simulink library "Course_Holes_Lib"  (R2025b)
settings: Solver=ode45  StartTime=0.0  StopTime=10.0  RelTol=1e-3  EnableMultiTasking=on
undefined symbols (not defined in the file): Mini_Golf_Param, X, Y, Z
libraries: Golf_Components_Lib x67, Contact_Forces_Lib x18, sm_lib x12
(part 1 of 2)
Description:
  | Copyright 2015-2025 The MathWorks, Inc.
settings Model: Creator=smiller  LastModifiedBy=smiller
settings SolverCC: AlgebraicLoopSolver=TrustRegion
settings DataIOCC: LimitDataPoints=on  SaveFormat=Array  SignalLoggingSaveFormat=ModelDataLogs  ReturnWorkspaceOutputs=off
settings OptimizationCC: ReuseModelBlockBuffer=off  ExpressionDepthLimit=2147483647.0  LifeSpan=inf
settings DebuggingCC: UnderspecifiedInitializationDetection=Classic  MergeDetectMultiDrivingBlocksExec=none  SolverPrmCheckMsg=warning  FcnCallInpInsideContextMsg=warning  UnconnectedInputMsg=warning  UnconnectedOutputMsg=warning  UnconnectedLineMsg=warning  AllowSymbolicDim=off  StateNameClashWarn=warning  PregeneratedLibrarySubsystemCodeDiagnostic=none  SFUnexpectedBacktrackingDiag=warning  SFNoUnconditionalDefaultTransitionDiag=warning  SFExecutionAtInitializationDiag=none  ArithmeticOperatorsInVariantConditions=warning
settings HardwareCC: ProdBitPerPointer=32.0  ProdBitPerSizeT=32.0  ProdBitPerPtrDiffT=32.0  ProdLargestAtomicFloat=None  ProdIntDivRoundTo=Undefined  ProdEndianess=Unspecified  ProdWordSize=32.0  ProdHWDeviceType=32-bit Generic
settings ModelReferenceCC: EnableRefExpFcnMdlSchedulingChecks=on  PropagateSignalLabelsOutOfModel=off
settings SFSimCC: SimUseLocalCustomCode=off  CustomCodeUndefinedFunction=UseInterfaceOnly
settings RTWCC: RTWUseLocalCustomCode=off  GPUComputeCapability=3.5  DLArmComputeVersion=19.05
settings CodeAppCC: StateflowObjectComments=on
settings GRTTargetCC: TargetLangStandard=C89/C90 (ANSI)
settings ConfigComp: CovMetricSettings=dw  CovSaveCumulativeToWorkspaceVar=on  CovSaveSingleToWorkspaceVar=on  CovExternalEMLEnable=off  CovSFcnEnable=off

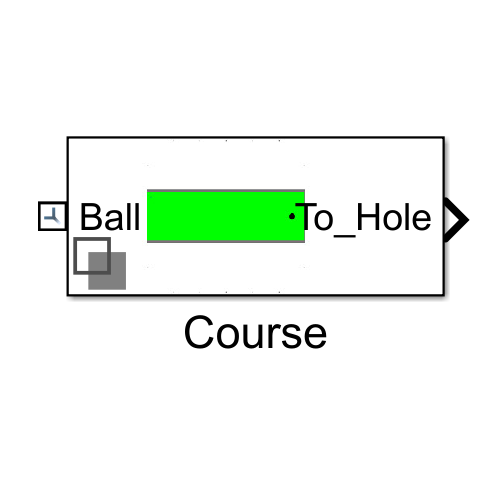
[thumbnail: Simulink's stored preview of the top-level diagram]
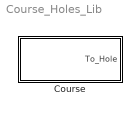
== system Course_Holes_Lib ==
  Course : Subsystem  Variant=on  VariantControlMode=label  LabelModeActiveChoice=Hole_1
      mask Display:
      | blk = CFL_activeVariantBlock(gcb);
      | eval(get_param(blk, 'MaskDisplay'));

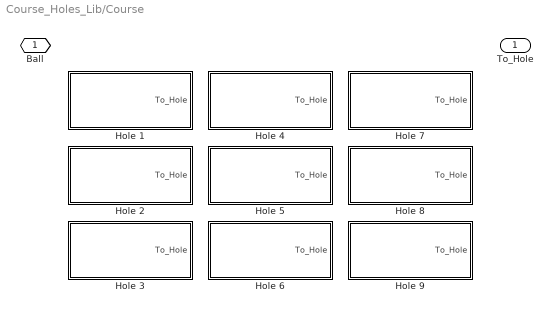
== system Course_Holes_Lib/Course ==
  Hole 1 : Subsystem  VariantControl=Hole_1
      mask Display: image(imread('Hole_1_IMAGE.jpg'));
  Hole 2 : Subsystem  VariantControl=Hole_2
      mask Display: image(imread('Hole_2_IMAGE.jpg'));
  Hole 3 : Subsystem  VariantControl=Hole_3
      mask Display: image(imread('Hole_3_IMAGE.jpg'));
  Hole 4 : Subsystem  VariantControl=Hole_4
      mask Display: image(imread('Hole_4_IMAGE.jpg'));
  Hole 5 : Subsystem  VariantControl=Hole_5
      mask Display: image(imread('Hole_5_IMAGE.jpg'));
  Hole 6 : Subsystem  VariantControl=Hole_6
      mask Display: image(imread('Hole_6_IMAGE.jpg'));
  Hole 7 : Subsystem  VariantControl=Hole_7
      mask Display: image(imread('Hole_7_IMAGE.jpg'));
  Hole 8 : Subsystem  VariantControl=Hole_8
      mask Display: image(imread('Hole_8_IMAGE.jpg'));
  Hole 9 : Subsystem  VariantControl=Hole_9
      mask Display: image(imread('Hole_9_IMAGE.jpg'));
  Ball : PMIOPort  Side=Left
  To_Hole : Outport  VectorParamsAs1DForOutWhenUnconnected=off

== system Course_Holes_Lib/Course/Hole 1 ==
  Back Wall : Golf_Components_Lib/Wall  length=Mini_Golf_Param.Hole_1.Wall_Back.Length  angle=Mini_Golf_Param.Hole_1.Wall_Back.Angle  offset=Mini_Golf_Param.Hole_1.Wall_Back.Offset  height=Mini_Golf_Param.Ball.Radius*2  width=Mini_Golf_Param.Wall.Width  wall_density=Mini_Golf_Param.Wall.Density  ball_radius=Mini_Golf_Param.Ball.Radius  contact_k=Mini_Golf_Param.Wall.Stiffness  contact_b=Mini_Golf_Param.Wall.Damping  low_pass_filt_const=Mini_Golf_Param.Wall.Low_Pass_Filt_Const
  Hole : Golf_Components_Lib/Hole  hole_offset=Mini_Golf_Param.Hole_1.Location  hole_radius=Mini_Golf_Param.Hole.Radius  hole_height=Mini_Golf_Param.Hole.Height  hole_stiffness=Mini_Golf_Param.Hole.Stiffness  hole_damping=Mini_Golf_Param.Hole.Damping  hole_deadzone=Mini_Golf_Param.Hole.Deadzone
  Left Wall : Golf_Components_Lib/Wall  length=Mini_Golf_Param.Hole_1.Wall_Left.Length  angle=Mini_Golf_Param.Hole_1.Wall_Left.Angle  offset=Mini_Golf_Param.Hole_1.Wall_Left.Offset  height=Mini_Golf_Param.Ball.Radius*2  width=Mini_Golf_Param.Wall.Width  wall_density=Mini_Golf_Param.Wall.Density  ball_radius=Mini_Golf_Param.Ball.Radius  contact_k=Mini_Golf_Param.Wall.Stiffness  contact_b=Mini_Golf_Param.Wall.Damping  low_pass_filt_const=Mini_Golf_Param.Wall.Low_Pass_Filt_Const
  Right Wall : Golf_Components_Lib/Wall  length=Mini_Golf_Param.Hole_1.Wall_Right.Length  angle=Mini_Golf_Param.Hole_1.Wall_Right.Angle  offset=Mini_Golf_Param.Hole_1.Wall_Right.Offset  height=Mini_Golf_Param.Ball.Radius*2  width=Mini_Golf_Param.Wall.Width  wall_density=Mini_Golf_Param.Wall.Density  ball_radius=Mini_Golf_Param.Ball.Radius  contact_k=Mini_Golf_Param.Wall.Stiffness  contact_b=Mini_Golf_Param.Wall.Damping  low_pass_filt_const=Mini_Golf_Param.Wall.Low_Pass_Filt_Const
  Surface : Golf_Components_Lib/Surface  width=Mini_Golf_Param.Hole_1.Surface_1.Width  length=Mini_Golf_Param.Hole_1.Surface_1.Length  offset=Mini_Golf_Param.Hole_1.Surface_1.Offset  height=Mini_Golf_Param.Surface_Height
  World Frame : sm_lib/Frames and Transforms/World Frame
  Ball : PMIOPort  Side=Left
  To_Hole : Outport  VectorParamsAs1DForOutWhenUnconnected=off
  wires:
  Hole/1 -> To_Hole/1
  connections:
  Surface/RConn1 -- World Frame/RConn1 -- Hole/RConn1 -- Left Wall/LConn1 -- Back Wall/LConn1 -- Right Wall/LConn1
  Hole/LConn1 -- Right Wall/RConn1 -- Back Wall/RConn1 -- Ball/RConn1 -- Left Wall/RConn1

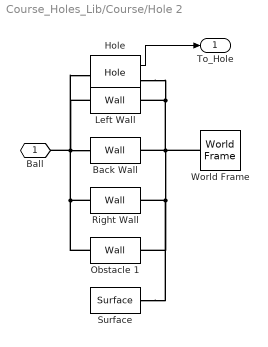
== system Course_Holes_Lib/Course/Hole 2 ==
  Back Wall : Golf_Components_Lib/Wall  length=Mini_Golf_Param.Hole_2.Wall_Back.Length  angle=Mini_Golf_Param.Hole_2.Wall_Back.Angle  offset=Mini_Golf_Param.Hole_2.Wall_Back.Offset  height=Mini_Golf_Param.Ball.Radius*2  width=Mini_Golf_Param.Wall.Width  wall_density=Mini_Golf_Param.Wall.Density  ball_radius=Mini_Golf_Param.Ball.Radius  contact_k=Mini_Golf_Param.Wall.Stiffness  contact_b=Mini_Golf_Param.Wall.Damping  low_pass_filt_const=Mini_Golf_Param.Wall.Low_Pass_Filt_Const
  Hole : Golf_Components_Lib/Hole  hole_offset=Mini_Golf_Param.Hole_2.Location  hole_radius=Mini_Golf_Param.Hole.Radius  hole_height=Mini_Golf_Param.Hole.Height  hole_stiffness=Mini_Golf_Param.Hole.Stiffness  hole_damping=Mini_Golf_Param.Hole.Damping  hole_deadzone=Mini_Golf_Param.Hole.Deadzone
  Left Wall : Golf_Components_Lib/Wall  length=Mini_Golf_Param.Hole_2.Wall_Left.Length  angle=Mini_Golf_Param.Hole_2.Wall_Left.Angle  offset=Mini_Golf_Param.Hole_2.Wall_Left.Offset  height=Mini_Golf_Param.Ball.Radius*2  width=Mini_Golf_Param.Wall.Width  wall_density=Mini_Golf_Param.Wall.Density  ball_radius=Mini_Golf_Param.Ball.Radius  contact_k=Mini_Golf_Param.Wall.Stiffness  contact_b=Mini_Golf_Param.Wall.Damping  low_pass_filt_const=Mini_Golf_Param.Wall.Low_Pass_Filt_Const
  Obstacle 1 : Golf_Components_Lib/Wall  length=Mini_Golf_Param.Hole_2.Wall_Obst1.Length  angle=Mini_Golf_Param.Hole_2.Wall_Obst1.Angle  offset=Mini_Golf_Param.Hole_2.Wall_Obst1.Offset  height=Mini_Golf_Param.Ball.Radius*2  width=Mini_Golf_Param.Wall.Width  wall_density=Mini_Golf_Param.Wall.Density  ball_radius=Mini_Golf_Param.Ball.Radius  contact_k=Mini_Golf_Param.Wall.Stiffness  contact_b=Mini_Golf_Param.Wall.Damping  low_pass_filt_const=Mini_Golf_Param.Wall.Low_Pass_Filt_Const
  Right Wall : Golf_Components_Lib/Wall  length=Mini_Golf_Param.Hole_2.Wall_Right.Length  angle=Mini_Golf_Param.Hole_2.Wall_Right.Angle  offset=Mini_Golf_Param.Hole_2.Wall_Right.Offset  height=Mini_Golf_Param.Ball.Radius*2  width=Mini_Golf_Param.Wall.Width  wall_density=Mini_Golf_Param.Wall.Density  ball_radius=Mini_Golf_Param.Ball.Radius  contact_k=Mini_Golf_Param.Wall.Stiffness  contact_b=Mini_Golf_Param.Wall.Damping  low_pass_filt_const=Mini_Golf_Param.Wall.Low_Pass_Filt_Const
  Surface : Golf_Components_Lib/Surface  width=Mini_Golf_Param.Hole_2.Surface_1.Width  length=Mini_Golf_Param.Hole_2.Surface_1.Length  offset=Mini_Golf_Param.Hole_2.Surface_1.Offset  height=Mini_Golf_Param.Surface_Height
  World Frame : sm_lib/Frames and Transforms/World Frame
  Ball : PMIOPort  Side=Left
  To_Hole : Outport  VectorParamsAs1DForOutWhenUnconnected=off
  wires:
  Hole/1 -> To_Hole/1
  connections:
  Right Wall/RConn1 -- Left Wall/RConn1 -- Hole/LConn1 -- Ball/RConn1 -- Back Wall/RConn1 -- Obstacle 1/RConn1
  World Frame/RConn1 -- Surface/RConn1 -- Obstacle 1/LConn1 -- Right Wall/LConn1 -- Back Wall/LConn1 -- Left Wall/LConn1 -- Hole/RConn1

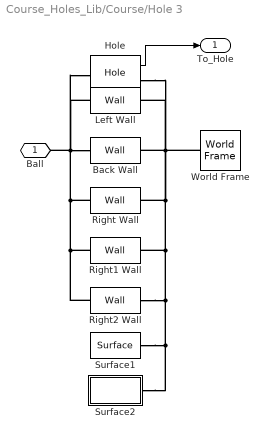
== system Course_Holes_Lib/Course/Hole 3 ==
  Back Wall : Golf_Components_Lib/Wall  length=Mini_Golf_Param.Hole_3.Wall_Back.Length  angle=Mini_Golf_Param.Hole_3.Wall_Back.Angle  offset=Mini_Golf_Param.Hole_3.Wall_Back.Offset  height=Mini_Golf_Param.Ball.Radius*2  width=Mini_Golf_Param.Wall.Width  wall_density=Mini_Golf_Param.Wall.Density  ball_radius=Mini_Golf_Param.Ball.Radius  contact_k=Mini_Golf_Param.Wall.Stiffness  contact_b=Mini_Golf_Param.Wall.Damping  low_pass_filt_const=Mini_Golf_Param.Wall.Low_Pass_Filt_Const
  Hole : Golf_Components_Lib/Hole  hole_offset=Mini_Golf_Param.Hole_3.Location  hole_radius=Mini_Golf_Param.Hole.Radius  hole_height=Mini_Golf_Param.Hole.Height  hole_stiffness=Mini_Golf_Param.Hole.Stiffness  hole_damping=Mini_Golf_Param.Hole.Damping  hole_deadzone=Mini_Golf_Param.Hole.Deadzone
  Left Wall : Golf_Components_Lib/Wall  length=Mini_Golf_Param.Hole_3.Wall_Left.Length  angle=Mini_Golf_Param.Hole_3.Wall_Left.Angle  offset=Mini_Golf_Param.Hole_3.Wall_Left.Offset  height=Mini_Golf_Param.Ball.Radius*2  width=Mini_Golf_Param.Wall.Width  wall_density=Mini_Golf_Param.Wall.Density  ball_radius=Mini_Golf_Param.Ball.Radius  contact_k=Mini_Golf_Param.Wall.Stiffness  contact_b=Mini_Golf_Param.Wall.Damping  low_pass_filt_const=Mini_Golf_Param.Wall.Low_Pass_Filt_Const
  Right Wall : Golf_Components_Lib/Wall  length=Mini_Golf_Param.Hole_3.Wall_Right.Length  angle=Mini_Golf_Param.Hole_3.Wall_Right.Angle  offset=Mini_Golf_Param.Hole_3.Wall_Right.Offset  height=Mini_Golf_Param.Ball.Radius*2  width=Mini_Golf_Param.Wall.Width  wall_density=Mini_Golf_Param.Wall.Density  ball_radius=Mini_Golf_Param.Ball.Radius  contact_k=Mini_Golf_Param.Wall.Stiffness  contact_b=Mini_Golf_Param.Wall.Damping  low_pass_filt_const=Mini_Golf_Param.Wall.Low_Pass_Filt_Const
  Right1 Wall : Golf_Components_Lib/Wall  length=Mini_Golf_Param.Hole_3.Wall_Right1.Length  angle=Mini_Golf_Param.Hole_3.Wall_Right1.Angle  offset=Mini_Golf_Param.Hole_3.Wall_Right1.Offset  height=Mini_Golf_Param.Ball.Radius*2  width=Mini_Golf_Param.Wall.Width  wall_density=Mini_Golf_Param.Wall.Density  ball_radius=Mini_Golf_Param.Ball.Radius  contact_k=Mini_Golf_Param.Wall.Stiffness  contact_b=Mini_Golf_Param.Wall.Damping  low_pass_filt_const=Mini_Golf_Param.Wall.Low_Pass_Filt_Const
  Right2 Wall : Golf_Components_Lib/Wall  length=Mini_Golf_Param.Hole_3.Wall_Right2.Length  angle=Mini_Golf_Param.Hole_3.Wall_Right2.Angle  offset=Mini_Golf_Param.Hole_3.Wall_Right2.Offset  height=Mini_Golf_Param.Ball.Radius*2  width=Mini_Golf_Param.Wall.Width  wall_density=Mini_Golf_Param.Wall.Density  ball_radius=Mini_Golf_Param.Ball.Radius  contact_k=Mini_Golf_Param.Wall.Stiffness  contact_b=Mini_Golf_Param.Wall.Damping  low_pass_filt_const=Mini_Golf_Param.Wall.Low_Pass_Filt_Const
  Surface1 : Golf_Components_Lib/Surface  width=Mini_Golf_Param.Hole_3.Surface_1.Width  length=Mini_Golf_Param.Hole_3.Surface_1.Length  offset=Mini_Golf_Param.Hole_3.Surface_1.Offset  height=Mini_Golf_Param.Surface_Height
  Surface2 : Subsystem  mask(Square Surface Patch for Golf Course){width=Mini_Golf_Param.Hole_3.Surface_2.Width, length=Mini_Golf_Param.Hole_3.Surface_2.Length, offset=Mini_Golf_Param.Hole_3.Surface_2.Offset, height=Mini_Golf_Param.Surface_Height}
      mask prompts: width "Surface Width (m)"; length "Surface Length (m)"; offset "Surface Offset (m)"; height "Surface Thickness(m)"
      mask help: Creates a square surface patch for golf course. All parameters are relative to the frame that is connected to the port.
  World Frame : sm_lib/Frames and Transforms/World Frame
  Ball : PMIOPort  Side=Left
  To_Hole : Outport  VectorParamsAs1DForOutWhenUnconnected=off
  wires:
  Hole/1 -> To_Hole/1
  connections:
  Surface1/RConn1 -- Surface2/RConn1 -- Right2 Wall/LConn1 -- Hole/RConn1 -- Left Wall/LConn1 -- Back Wall/LConn1 -- World Frame/RConn1 -- Right Wall/LConn1 -- Right1 Wall/LConn1
  Right1 Wall/RConn1 -- Right2 Wall/RConn1 -- Back Wall/RConn1 -- Ball/RConn1 -- Hole/LConn1 -- Left Wall/RConn1 -- Right Wall/RConn1

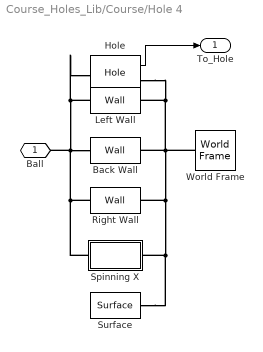
== system Course_Holes_Lib/Course/Hole 4 ==
  Back Wall : Golf_Components_Lib/Wall  length=Mini_Golf_Param.Hole_1.Wall_Back.Length  angle=Mini_Golf_Param.Hole_1.Wall_Back.Angle  offset=Mini_Golf_Param.Hole_1.Wall_Back.Offset  height=Mini_Golf_Param.Ball.Radius*2  width=Mini_Golf_Param.Wall.Width  wall_density=Mini_Golf_Param.Wall.Density  ball_radius=Mini_Golf_Param.Ball.Radius  contact_k=Mini_Golf_Param.Wall.Stiffness  contact_b=Mini_Golf_Param.Wall.Damping  low_pass_filt_const=Mini_Golf_Param.Wall.Low_Pass_Filt_Const
  Hole : Golf_Components_Lib/Hole  hole_offset=Mini_Golf_Param.Hole_1.Location  hole_radius=Mini_Golf_Param.Hole.Radius  hole_height=Mini_Golf_Param.Hole.Height  hole_stiffness=Mini_Golf_Param.Hole.Stiffness  hole_damping=Mini_Golf_Param.Hole.Damping  hole_deadzone=Mini_Golf_Param.Hole.Deadzone
  Left Wall : Golf_Components_Lib/Wall  length=Mini_Golf_Param.Hole_1.Wall_Left.Length  angle=Mini_Golf_Param.Hole_1.Wall_Left.Angle  offset=Mini_Golf_Param.Hole_1.Wall_Left.Offset  height=Mini_Golf_Param.Ball.Radius*2  width=Mini_Golf_Param.Wall.Width  wall_density=Mini_Golf_Param.Wall.Density  ball_radius=Mini_Golf_Param.Ball.Radius  contact_k=Mini_Golf_Param.Wall.Stiffness  contact_b=Mini_Golf_Param.Wall.Damping  low_pass_filt_const=Mini_Golf_Param.Wall.Low_Pass_Filt_Const
  Right Wall : Golf_Components_Lib/Wall  length=Mini_Golf_Param.Hole_1.Wall_Right.Length  angle=Mini_Golf_Param.Hole_1.Wall_Right.Angle  offset=Mini_Golf_Param.Hole_1.Wall_Right.Offset  height=Mini_Golf_Param.Ball.Radius*2  width=Mini_Golf_Param.Wall.Width  wall_density=Mini_Golf_Param.Wall.Density  ball_radius=Mini_Golf_Param.Ball.Radius  contact_k=Mini_Golf_Param.Wall.Stiffness  contact_b=Mini_Golf_Param.Wall.Damping  low_pass_filt_const=Mini_Golf_Param.Wall.Low_Pass_Filt_Const
  Spinning X : Subsystem
  Surface : Golf_Components_Lib/Surface  width=Mini_Golf_Param.Hole_4.Surface_1.Width  length=Mini_Golf_Param.Hole_4.Surface_1.Length  offset=Mini_Golf_Param.Hole_4.Surface_1.Offset  height=Mini_Golf_Param.Surface_Height
  World Frame : sm_lib/Frames and Transforms/World Frame
  Ball : PMIOPort  Side=Left
  To_Hole : Outport  VectorParamsAs1DForOutWhenUnconnected=off
  wires:
  Hole/1 -> To_Hole/1
  connections:
  Spinning X/LConn1 -- Right Wall/RConn1 -- Left Wall/RConn1 -- Hole/LConn1 -- Ball/RConn1 -- Back Wall/RConn1
  Back Wall/LConn1 -- Left Wall/LConn1 -- Hole/RConn1 -- World Frame/RConn1 -- Right Wall/LConn1 -- Spinning X/RConn1 -- Surface/RConn1

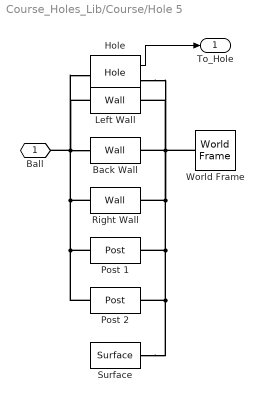
== system Course_Holes_Lib/Course/Hole 5 ==
  Back Wall : Golf_Components_Lib/Wall  length=Mini_Golf_Param.Hole_5.Wall_Back.Length  angle=Mini_Golf_Param.Hole_5.Wall_Back.Angle  offset=Mini_Golf_Param.Hole_5.Wall_Back.Offset  height=Mini_Golf_Param.Ball.Radius*2  width=Mini_Golf_Param.Wall.Width  wall_density=Mini_Golf_Param.Wall.Density  ball_radius=Mini_Golf_Param.Ball.Radius  contact_k=Mini_Golf_Param.Wall.Stiffness  contact_b=Mini_Golf_Param.Wall.Damping  low_pass_filt_const=Mini_Golf_Param.Wall.Low_Pass_Filt_Const
  Hole : Golf_Components_Lib/Hole  hole_offset=Mini_Golf_Param.Hole_5.Location  hole_radius=Mini_Golf_Param.Hole.Radius  hole_height=Mini_Golf_Param.Hole.Height  hole_stiffness=Mini_Golf_Param.Hole.Stiffness  hole_damping=Mini_Golf_Param.Hole.Damping  hole_deadzone=Mini_Golf_Param.Hole.Deadzone
  Left Wall : Golf_Components_Lib/Wall  length=Mini_Golf_Param.Hole_5.Wall_Left.Length  angle=Mini_Golf_Param.Hole_5.Wall_Left.Angle  offset=Mini_Golf_Param.Hole_5.Wall_Left.Offset  height=Mini_Golf_Param.Ball.Radius*2  width=Mini_Golf_Param.Wall.Width  wall_density=Mini_Golf_Param.Wall.Density  ball_radius=Mini_Golf_Param.Ball.Radius  contact_k=Mini_Golf_Param.Wall.Stiffness  contact_b=Mini_Golf_Param.Wall.Damping  low_pass_filt_const=Mini_Golf_Param.Wall.Low_Pass_Filt_Const
  Post 1 : Golf_Components_Lib/Post  width=Mini_Golf_Param.Hole_5.Post_1.Diameter  height=Mini_Golf_Param.Ball.Radius*2  offset=Mini_Golf_Param.Hole_5.Post_1.Offset  ball_radius=Mini_Golf_Param.Ball.Radius  contact_k=Mini_Golf_Param.Wall.Stiffness  contact_b=Mini_Golf_Param.Wall.Damping  low_pass_filt_const=Mini_Golf_Param.Wall.Low_Pass_Filt_Const
  Post 2 : Golf_Components_Lib/Post  width=Mini_Golf_Param.Hole_5.Post_2.Diameter  height=Mini_Golf_Param.Ball.Radius*2  offset=Mini_Golf_Param.Hole_5.Post_2.Offset  ball_radius=Mini_Golf_Param.Ball.Radius  contact_k=Mini_Golf_Param.Wall.Stiffness  contact_b=Mini_Golf_Param.Wall.Damping  low_pass_filt_const=Mini_Golf_Param.Wall.Low_Pass_Filt_Const
  Right Wall : Golf_Components_Lib/Wall  length=Mini_Golf_Param.Hole_5.Wall_Right.Length  angle=Mini_Golf_Param.Hole_5.Wall_Right.Angle  offset=Mini_Golf_Param.Hole_5.Wall_Right.Offset  height=Mini_Golf_Param.Ball.Radius*2  width=Mini_Golf_Param.Wall.Width  wall_density=Mini_Golf_Param.Wall.Density  ball_radius=Mini_Golf_Param.Ball.Radius  contact_k=Mini_Golf_Param.Wall.Stiffness  contact_b=Mini_Golf_Param.Wall.Damping  low_pass_filt_const=Mini_Golf_Param.Wall.Low_Pass_Filt_Const
  Surface : Golf_Components_Lib/Surface  width=Mini_Golf_Param.Hole_5.Surface_1.Width  length=Mini_Golf_Param.Hole_5.Surface_1.Length  offset=Mini_Golf_Param.Hole_5.Surface_1.Offset  height=Mini_Golf_Param.Surface_Height
  World Frame : sm_lib/Frames and Transforms/World Frame
  Ball : PMIOPort  Side=Left
  To_Hole : Outport  VectorParamsAs1DForOutWhenUnconnected=off
  wires:
  Hole/1 -> To_Hole/1
  connections:
  Post 1/RConn1 -- Right Wall/RConn1 -- Left Wall/RConn1 -- Hole/LConn1 -- Ball/RConn1 -- Back Wall/RConn1 -- Post 2/RConn1
  Surface/RConn1 -- Post 1/LConn1 -- Back Wall/LConn1 -- Left Wall/LConn1 -- Hole/RConn1 -- World Frame/RConn1 -- Right Wall/LConn1 -- Post 2/LConn1

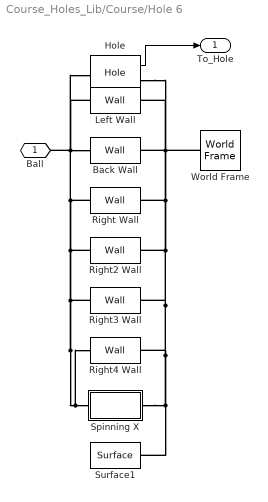
== system Course_Holes_Lib/Course/Hole 6 ==
  Back Wall : Golf_Components_Lib/Wall  length=Mini_Golf_Param.Hole_6.Wall_Back.Length  angle=Mini_Golf_Param.Hole_6.Wall_Back.Angle  offset=Mini_Golf_Param.Hole_6.Wall_Back.Offset  height=Mini_Golf_Param.Ball.Radius*2  width=Mini_Golf_Param.Wall.Width  wall_density=Mini_Golf_Param.Wall.Density  ball_radius=Mini_Golf_Param.Ball.Radius  contact_k=Mini_Golf_Param.Wall.Stiffness  contact_b=Mini_Golf_Param.Wall.Damping  low_pass_filt_const=Mini_Golf_Param.Wall.Low_Pass_Filt_Const
  Hole : Golf_Components_Lib/Hole  hole_offset=Mini_Golf_Param.Hole_6.Location  hole_radius=Mini_Golf_Param.Hole.Radius  hole_height=Mini_Golf_Param.Hole.Height  hole_stiffness=Mini_Golf_Param.Hole.Stiffness  hole_damping=Mini_Golf_Param.Hole.Damping  hole_deadzone=Mini_Golf_Param.Hole.Deadzone
  Left Wall : Golf_Components_Lib/Wall  length=Mini_Golf_Param.Hole_6.Wall_Left.Length  angle=Mini_Golf_Param.Hole_6.Wall_Left.Angle  offset=Mini_Golf_Param.Hole_6.Wall_Left.Offset  height=Mini_Golf_Param.Ball.Radius*2  width=Mini_Golf_Param.Wall.Width  wall_density=Mini_Golf_Param.Wall.Density  ball_radius=Mini_Golf_Param.Ball.Radius  contact_k=Mini_Golf_Param.Wall.Stiffness  contact_b=Mini_Golf_Param.Wall.Damping  low_pass_filt_const=Mini_Golf_Param.Wall.Low_Pass_Filt_Const
  Right Wall : Golf_Components_Lib/Wall  length=Mini_Golf_Param.Hole_6.Wall_Right.Length  angle=Mini_Golf_Param.Hole_6.Wall_Right.Angle  offset=Mini_Golf_Param.Hole_6.Wall_Right.Offset  height=Mini_Golf_Param.Ball.Radius*2  width=Mini_Golf_Param.Wall.Width  wall_density=Mini_Golf_Param.Wall.Density  ball_radius=Mini_Golf_Param.Ball.Radius  contact_k=Mini_Golf_Param.Wall.Stiffness  contact_b=Mini_Golf_Param.Wall.Damping  low_pass_filt_const=Mini_Golf_Param.Wall.Low_Pass_Filt_Const
  Right2 Wall : Golf_Components_Lib/Wall  length=Mini_Golf_Param.Hole_6.Wall_Right2.Length  angle=Mini_Golf_Param.Hole_6.Wall_Right2.Angle  offset=Mini_Golf_Param.Hole_6.Wall_Right2.Offset  height=Mini_Golf_Param.Ball.Radius*2  width=Mini_Golf_Param.Wall.Width  wall_density=Mini_Golf_Param.Wall.Density  ball_radius=Mini_Golf_Param.Ball.Radius  contact_k=Mini_Golf_Param.Wall.Stiffness  contact_b=Mini_Golf_Param.Wall.Damping  low_pass_filt_const=Mini_Golf_Param.Wall.Low_Pass_Filt_Const
  Right3 Wall : Golf_Components_Lib/Wall  length=Mini_Golf_Param.Hole_6.Wall_Right3.Length  angle=Mini_Golf_Param.Hole_6.Wall_Right3.Angle  offset=Mini_Golf_Param.Hole_6.Wall_Right3.Offset  height=Mini_Golf_Param.Ball.Radius*2  width=Mini_Golf_Param.Wall.Width  wall_density=Mini_Golf_Param.Wall.Density  ball_radius=Mini_Golf_Param.Ball.Radius  contact_k=Mini_Golf_Param.Wall.Stiffness  contact_b=Mini_Golf_Param.Wall.Damping  low_pass_filt_const=Mini_Golf_Param.Wall.Low_Pass_Filt_Const
  Right4 Wall : Golf_Components_Lib/Wall  length=Mini_Golf_Param.Hole_6.Wall_Right4.Length  angle=Mini_Golf_Param.Hole_6.Wall_Right4.Angle  offset=Mini_Golf_Param.Hole_6.Wall_Right4.Offset  height=Mini_Golf_Param.Ball.Radius*2  width=Mini_Golf_Param.Wall.Width  wall_density=Mini_Golf_Param.Wall.Density  ball_radius=Mini_Golf_Param.Ball.Radius  contact_k=Mini_Golf_Param.Wall.Stiffness  contact_b=Mini_Golf_Param.Wall.Damping  low_pass_filt_const=Mini_Golf_Param.Wall.Low_Pass_Filt_Const
  Spinning X : Subsystem
  Surface1 : Golf_Components_Lib/Surface  width=Mini_Golf_Param.Hole_6.Surface_1.Width  length=Mini_Golf_Param.Hole_6.Surface_1.Length  offset=Mini_Golf_Param.Hole_6.Surface_1.Offset  height=Mini_Golf_Param.Surface_Height
  World Frame : sm_lib/Frames and Transforms/World Frame
  Ball : PMIOPort  Side=Left
  To_Hole : Outport  VectorParamsAs1DForOutWhenUnconnected=off
  wires:
  Hole/1 -> To_Hole/1
  connections:
  Spinning X/LConn1 -- Right3 Wall/RConn1 -- Right2 Wall/RConn1 -- Right Wall/RConn1 -- Left Wall/RConn1 -- Hole/LConn1 -- Ball/RConn1 -- Back Wall/RConn1 -- Right4 Wall/RConn1
  Spinning X/RConn1 -- Right2 Wall/LConn1 -- Right Wall/LConn1 -- World Frame/RConn1 -- Back Wall/LConn1 -- Left Wall/LConn1 -- Hole/RConn1 -- Right3 Wall/LConn1 -- Right4 Wall/LConn1 -- Surface1/RConn1

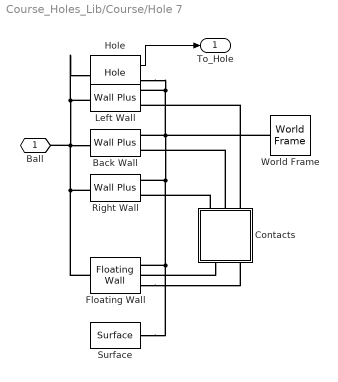
== system Course_Holes_Lib/Course/Hole 7 ==
  Back Wall : Golf_Components_Lib/Wall Plus  length=Mini_Golf_Param.Hole_7.Wall_Back.Length  angle=Mini_Golf_Param.Hole_7.Wall_Back.Angle  offset=Mini_Golf_Param.Hole_7.Wall_Back.Offset  height=Mini_Golf_Param.Ball.Radius*2  width=Mini_Golf_Param.Wall.Width  ball_radius=Mini_Golf_Param.Ball.Radius  contact_k=Mini_Golf_Param.Wall.Stiffness  contact_b=Mini_Golf_Param.Wall.Damping  low_pass_filt_const=Mini_Golf_Param.Wall.Low_Pass_Filt_Const
  Contacts : Subsystem
  Floating Wall : Golf_Components_Lib/Floating Wall  length=Mini_Golf_Param.Hole_7.Wall_Obst1.Length  angle=Mini_Golf_Param.Hole_7.Wall_Obst1.Angle  offset=Mini_Golf_Param.Hole_7.Wall_Obst1.Offset  height=Mini_Golf_Param.Ball.Radius*2  width=Mini_Golf_Param.Wall.Width  wall_friction=Mini_Golf_Param.Hole_7.Wall_Obst1.Friction  wall_rot_friction=Mini_Golf_Param.Hole_7.Wall_Obst1.Rot_Friction  ball_radius=Mini_Golf_Param.Ball.Radius  contact_k=Mini_Golf_Param.Wall.Stiffness  contact_b=Mini_Golf_Param.Wall.Damping  low_pass_filt_const=Mini_Golf_Param.Wall.Low_Pass_Filt_Const
  Hole : Golf_Components_Lib/Hole  hole_offset=Mini_Golf_Param.Hole_7.Location  hole_radius=Mini_Golf_Param.Hole.Radius  hole_height=Mini_Golf_Param.Hole.Height  hole_stiffness=Mini_Golf_Param.Hole.Stiffness  hole_damping=Mini_Golf_Param.Hole.Damping  hole_deadzone=Mini_Golf_Param.Hole.Deadzone
  Left Wall : Golf_Components_Lib/Wall Plus  length=Mini_Golf_Param.Hole_7.Wall_Left.Length  angle=Mini_Golf_Param.Hole_7.Wall_Left.Angle  offset=Mini_Golf_Param.Hole_7.Wall_Left.Offset  height=Mini_Golf_Param.Ball.Radius*2  width=Mini_Golf_Param.Wall.Width  ball_radius=Mini_Golf_Param.Ball.Radius  contact_k=Mini_Golf_Param.Wall.Stiffness  contact_b=Mini_Golf_Param.Wall.Damping  low_pass_filt_const=Mini_Golf_Param.Wall.Low_Pass_Filt_Const
  Right Wall : Golf_Components_Lib/Wall Plus  length=Mini_Golf_Param.Hole_7.Wall_Right.Length  angle=Mini_Golf_Param.Hole_7.Wall_Right.Angle  offset=Mini_Golf_Param.Hole_7.Wall_Right.Offset  height=Mini_Golf_Param.Ball.Radius*2  width=Mini_Golf_Param.Wall.Width  ball_radius=Mini_Golf_Param.Ball.Radius  contact_k=Mini_Golf_Param.Wall.Stiffness  contact_b=Mini_Golf_Param.Wall.Damping  low_pass_filt_const=Mini_Golf_Param.Wall.Low_Pass_Filt_Const
  Surface : Golf_Components_Lib/Surface  width=Mini_Golf_Param.Hole_7.Surface_1.Width  length=Mini_Golf_Param.Hole_7.Surface_1.Length  offset=Mini_Golf_Param.Hole_7.Surface_1.Offset  height=Mini_Golf_Param.Surface_Height
  World Frame : sm_lib/Frames and Transforms/World Frame
  Ball : PMIOPort  Side=Left
  To_Hole : Outport  VectorParamsAs1DForOutWhenUnconnected=off
  wires:
  Hole/1 -> To_Hole/1
  connections:
  Right Wall/LConn1 -- Hole/RConn1 -- Left Wall/LConn1 -- World Frame/RConn1 -- Back Wall/LConn1 -- Surface/RConn1 -- Floating Wall/LConn1
  Ball/RConn1 -- Floating Wall/RConn1 -- Right Wall/RConn1 -- Hole/LConn1 -- Left Wall/RConn1 -- Back Wall/RConn1
  Contacts/LConn1 -- Floating Wall/LConn2
  Floating Wall/LConn3 -- Contacts/LConn2
  Contacts/RConn1 -- Right Wall/LConn2
  Contacts/RConn2 -- Back Wall/LConn2
  Contacts/RConn3 -- Left Wall/LConn2

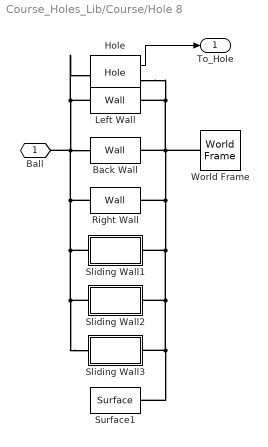
== system Course_Holes_Lib/Course/Hole 8 ==
  Back Wall : Golf_Components_Lib/Wall  length=Mini_Golf_Param.Hole_8.Wall_Back.Length  angle=Mini_Golf_Param.Hole_8.Wall_Back.Angle  offset=Mini_Golf_Param.Hole_8.Wall_Back.Offset  height=Mini_Golf_Param.Ball.Radius*2  width=Mini_Golf_Param.Wall.Width  wall_density=Mini_Golf_Param.Wall.Density  ball_radius=Mini_Golf_Param.Ball.Radius  contact_k=Mini_Golf_Param.Wall.Stiffness  contact_b=Mini_Golf_Param.Wall.Damping  low_pass_filt_const=Mini_Golf_Param.Wall.Low_Pass_Filt_Const
  Hole : Golf_Components_Lib/Hole  hole_offset=Mini_Golf_Param.Hole_8.Location  hole_radius=Mini_Golf_Param.Hole.Radius  hole_height=Mini_Golf_Param.Hole.Height  hole_stiffness=Mini_Golf_Param.Hole.Stiffness  hole_damping=Mini_Golf_Param.Hole.Damping  hole_deadzone=Mini_Golf_Param.Hole.Deadzone
  Left Wall : Golf_Components_Lib/Wall  length=Mini_Golf_Param.Hole_8.Wall_Left.Length  angle=Mini_Golf_Param.Hole_8.Wall_Left.Angle  offset=Mini_Golf_Param.Hole_8.Wall_Left.Offset  height=Mini_Golf_Param.Ball.Radius*2  width=Mini_Golf_Param.Wall.Width  wall_density=Mini_Golf_Param.Wall.Density  ball_radius=Mini_Golf_Param.Ball.Radius  contact_k=Mini_Golf_Param.Wall.Stiffness  contact_b=Mini_Golf_Param.Wall.Damping  low_pass_filt_const=Mini_Golf_Param.Wall.Low_Pass_Filt_Const
  Right Wall : Golf_Components_Lib/Wall  length=Mini_Golf_Param.Hole_8.Wall_Right.Length  angle=Mini_Golf_Param.Hole_8.Wall_Right.Angle  offset=Mini_Golf_Param.Hole_8.Wall_Right.Offset  height=Mini_Golf_Param.Ball.Radius*2  width=Mini_Golf_Param.Wall.Width  wall_density=Mini_Golf_Param.Wall.Density  ball_radius=Mini_Golf_Param.Ball.Radius  contact_k=Mini_Golf_Param.Wall.Stiffness  contact_b=Mini_Golf_Param.Wall.Damping  low_pass_filt_const=Mini_Golf_Param.Wall.Low_Pass_Filt_Const
  Sliding Wall1 : Subsystem
  Sliding Wall2 : Subsystem
  Sliding Wall3 : Subsystem
  Surface1 : Golf_Components_Lib/Surface  width=Mini_Golf_Param.Hole_8.Surface_1.Width  length=Mini_Golf_Param.Hole_8.Surface_1.Length  offset=Mini_Golf_Param.Hole_8.Surface_1.Offset  height=Mini_Golf_Param.Surface_Height
  World Frame : sm_lib/Frames and Transforms/World Frame
  Ball : PMIOPort  Side=Left
  To_Hole : Outport  VectorParamsAs1DForOutWhenUnconnected=off
  wires:
  Hole/1 -> To_Hole/1
  connections:
  Sliding Wall3/LConn1 -- Surface1/RConn1 -- Hole/RConn1 -- Left Wall/LConn1 -- Back Wall/LConn1 -- World Frame/RConn1 -- Right Wall/LConn1 -- Sliding Wall1/LConn1 -- Sliding Wall2/LConn1
  Sliding Wall3/RConn1 -- Back Wall/RConn1 -- Ball/RConn1 -- Hole/LConn1 -- Left Wall/RConn1 -- Right Wall/RConn1 -- Sliding Wall1/RConn1 -- Sliding Wall2/RConn1

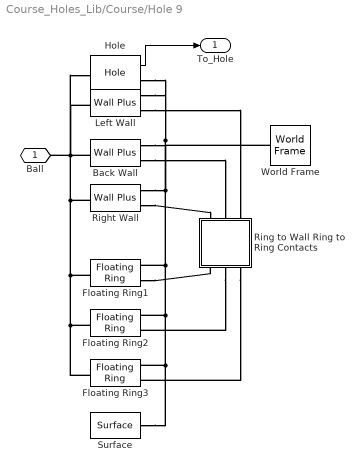
== system Course_Holes_Lib/Course/Hole 9 ==
  Back Wall : Golf_Components_Lib/Wall Plus  length=Mini_Golf_Param.Hole_9.Wall_Back.Length  angle=Mini_Golf_Param.Hole_9.Wall_Back.Angle  offset=Mini_Golf_Param.Hole_9.Wall_Back.Offset  height=Mini_Golf_Param.Ball.Radius*2  width=Mini_Golf_Param.Wall.Width  ball_radius=Mini_Golf_Param.Ball.Radius  contact_k=Mini_Golf_Param.Wall.Stiffness  contact_b=Mini_Golf_Param.Wall.Damping  low_pass_filt_const=Mini_Golf_Param.Wall.Low_Pass_Filt_Const
  Floating Ring1 : Golf_Components_Lib/Floating Ring  extr_xy_data=Mini_Golf_Param.Hole_9.Extr1.Cross_Section_Data  offset=Mini_Golf_Param.Hole_9.Extr1.Offset  height=Mini_Golf_Param.Ball.Radius*2  diameter=Mini_Golf_Param.Hole_9.Extr1.Ring_Outer_Diameter  extr1_friction=Mini_Golf_Param.Hole_9.Extr1.Friction  ball_radius=Mini_Golf_Param.Ball.Radius  contact_k=Mini_Golf_Param.Wall.Stiffness  contact_b=Mini_Golf_Param.Wall.Damping  low_pass_filt_const=Mini_Golf_Param.Wall.Low_Pass_Filt_Const
  Floating Ring2 : Golf_Components_Lib/Floating Ring  extr_xy_data=Mini_Golf_Param.Hole_9.Extr2.Cross_Section_Data  offset=Mini_Golf_Param.Hole_9.Extr2.Offset  height=Mini_Golf_Param.Ball.Radius*2  diameter=Mini_Golf_Param.Hole_9.Extr2.Ring_Outer_Diameter  extr1_friction=Mini_Golf_Param.Hole_9.Extr2.Friction  ball_radius=Mini_Golf_Param.Ball.Radius  contact_k=Mini_Golf_Param.Wall.Stiffness  contact_b=Mini_Golf_Param.Wall.Damping  low_pass_filt_const=Mini_Golf_Param.Wall.Low_Pass_Filt_Const
  Floating Ring3 : Golf_Components_Lib/Floating Ring  extr_xy_data=Mini_Golf_Param.Hole_9.Extr3.Cross_Section_Data  offset=Mini_Golf_Param.Hole_9.Extr3.Offset  height=Mini_Golf_Param.Ball.Radius*2  diameter=Mini_Golf_Param.Hole_9.Extr3.Ring_Outer_Diameter  extr1_friction=Mini_Golf_Param.Hole_9.Extr3.Friction  ball_radius=Mini_Golf_Param.Ball.Radius  contact_k=Mini_Golf_Param.Wall.Stiffness  contact_b=Mini_Golf_Param.Wall.Damping  low_pass_filt_const=Mini_Golf_Param.Wall.Low_Pass_Filt_Const
  Hole : Golf_Components_Lib/Hole  hole_offset=Mini_Golf_Param.Hole_9.Location  hole_radius=Mini_Golf_Param.Hole.Radius  hole_height=Mini_Golf_Param.Hole.Height  hole_stiffness=Mini_Golf_Param.Hole.Stiffness  hole_damping=Mini_Golf_Param.Hole.Damping  hole_deadzone=Mini_Golf_Param.Hole.Deadzone
  Left Wall : Golf_Components_Lib/Wall Plus  length=Mini_Golf_Param.Hole_9.Wall_Left.Length  angle=Mini_Golf_Param.Hole_9.Wall_Left.Angle  offset=Mini_Golf_Param.Hole_9.Wall_Left.Offset  height=Mini_Golf_Param.Ball.Radius*2  width=Mini_Golf_Param.Wall.Width  ball_radius=Mini_Golf_Param.Ball.Radius  contact_k=Mini_Golf_Param.Wall.Stiffness  contact_b=Mini_Golf_Param.Wall.Damping  low_pass_filt_const=Mini_Golf_Param.Wall.Low_Pass_Filt_Const
  Right Wall : Golf_Components_Lib/Wall Plus  length=Mini_Golf_Param.Hole_9.Wall_Right.Length  angle=Mini_Golf_Param.Hole_9.Wall_Right.Angle  offset=Mini_Golf_Param.Hole_9.Wall_Right.Offset  height=Mini_Golf_Param.Ball.Radius*2  width=Mini_Golf_Param.Wall.Width  ball_radius=Mini_Golf_Param.Ball.Radius  contact_k=Mini_Golf_Param.Wall.Stiffness  contact_b=Mini_Golf_Param.Wall.Damping  low_pass_filt_const=Mini_Golf_Param.Wall.Low_Pass_Filt_Const
  Ring to Wall Ring to Ring Contacts : Subsystem
  Surface : Golf_Components_Lib/Surface  width=Mini_Golf_Param.Hole_9.Surface_1.Width  length=Mini_Golf_Param.Hole_9.Surface_1.Length  offset=Mini_Golf_Param.Hole_9.Surface_1.Offset  height=Mini_Golf_Param.Surface_Height
  World Frame : sm_lib/Frames and Transforms/World Frame
  Ball : PMIOPort  Side=Left
  To_Hole : Outport  VectorParamsAs1DForOutWhenUnconnected=off
  wires:
  Hole/1 -> To_Hole/1
  connections:
  Left Wall/LConn2 -- Ring to Wall Ring to Ring Contacts/RConn3
  Back Wall/LConn2 -- Ring to Wall Ring to Ring Contacts/RConn2
  Right Wall/LConn2 -- Ring to Wall Ring to Ring Contacts/RConn1
  Floating Ring1/LConn2 -- Ring to Wall Ring to Ring Contacts/LConn1
  Floating Ring2/RConn1 -- Floating Ring1/RConn1 -- Right Wall/RConn1 -- Back Wall/RConn1 -- Left Wall/RConn1 -- Hole/LConn1 -- Ball/RConn1 -- Floating Ring3/RConn1
  Surface/RConn1 -- Right Wall/LConn1 -- Back Wall/LConn1 -- World Frame/RConn1 -- Left Wall/LConn1 -- Hole/RConn1 -- Floating Ring1/LConn1 -- Floating Ring2/LConn1 -- Floating Ring3/LConn1
  Ring to Wall Ring to Ring Contacts/LConn2 -- Floating Ring2/LConn2
  Ring to Wall Ring to Ring Contacts/LConn3 -- Floating Ring3/LConn2

== system Course_Holes_Lib/Course/Hole 3/Surface2 ==
  Rigid Transform : sm_lib/Frames and Transforms/Rigid Transform  RotationMethod=None  FollAlignAxisA=+X  BaseAlignAxisA=+Y  FollAlignAxisB=+Y  BaseAlignAxisB=+Z  RotationStandardAxis=+Z  RotationAngle=0  RotationAngleUnits=deg  RotationArbitraryAxis=[0 0 1]  RotationSequenceAxes=FollowerAxes  RotationSequence=XYX  RotationSequenceAngles=[0 0 0]  RotationSequenceAnglesUnits=deg  RotationMatrix=[1 0 0; 0 1 0; 0 0 1]  Quaternion=[1 0 0 0]  TranslationMethod=Cartesian  TranslationCartesianOffset=offset  TranslationCartesianOffsetUnits=m  TranslationStandardAxis=+Z  TranslationStandardOffset=0  TranslationStandardOffsetUnits=m  TranslationROffset=0  TranslationROffsetUnits=m  TranslationThetaOffset=0  TranslationThetaOffsetUnits=deg  TranslationZOffset=0  TranslationZOffsetUnits=m
  Surface Patch : sm_lib/Body Elements/Brick Solid  BrickDimensions=[length width height]  BrickDimensionsUnits=m  ExportEntireGeometry=off  InertiaType=CalculateFromGeometry  BasedOnType=Density  Density=1  DensityUnits=kg/(m^3)  Mass=1  MassUnits=kg  CenterOfMass=[0 0 0]  CenterOfMassUnits=m  MomentsOfInertia=[1 1 1]  MomentsOfInertiaUnits=kg*m^2  ProductsOfInertia=[0 0 0]  ProductsOfInertiaUnits=kg*m^2  GraphicType=FromGeometry  MarkerShape=Sphere  MarkerSize=10  GraphicVisPropType=SimpleVisualProperties  GraphicDiffuseColor=[0.0 0.8 0.2]  GraphicOpacity=1.0  GraphicSpecularColor=[0.5 0.5 0.5 1.0]  GraphicAmbientColor=[0.15 0.15 0.15 1.0]  GraphicEmissiveColor=[0.0 0.0 0.0 1.0]  GraphicShininess=75  DoExposeReferenceFrame=on  SerializedFrames=<Frames/>
  Weld Joint : sm_lib/Joints/Weld Joint  JointMode=Normal  CompositeWrenchDir=FollowerOnBase  CompositeWrenchFrame=BaseFrame  SenseConstraintForce=off  SenseConstraintTorque=off  SenseTotalForce=off  SenseTotalTorque=off
  Ref : PMIOPort  Side=Right
  connections:
  Weld Joint/LConn1 -- Ref/RConn1
  Rigid Transform/LConn1 -- Weld Joint/RConn1
  Rigid Transform/RConn1 -- Surface Patch/RConn1

== system Course_Holes_Lib/Course/Hole 4/Spinning X ==
  Spinning Wall : Golf_Components_Lib/Spinning Wall  length=Mini_Golf_Param.Hole_4.Wall_Obst1.Length  angle=Mini_Golf_Param.Hole_4.Wall_Obst1.Angle  offset=Mini_Golf_Param.Hole_4.Wall_Obst1.Offset  ang_spd=Mini_Golf_Param.Hole_4.Obst_Pin.Speed  height=Mini_Golf_Param.Ball.Radius*2  width=Mini_Golf_Param.Wall.Width  wall_density=Mini_Golf_Param.Wall.Density  ball_radius=Mini_Golf_Param.Ball.Radius  contact_k=Mini_Golf_Param.Wall.Stiffness  contact_b=Mini_Golf_Param.Wall.Damping  low_pass_filt_const=Mini_Golf_Param.Wall.Low_Pass_Filt_Const
  Wall : Golf_Components_Lib/Wall  length=Mini_Golf_Param.Hole_4.Wall_Obst2.Length  angle=Mini_Golf_Param.Hole_4.Wall_Obst2.Angle  offset=Mini_Golf_Param.Hole_4.Wall_Obst2.Offset*0  height=Mini_Golf_Param.Ball.Radius*2  width=Mini_Golf_Param.Wall.Width  wall_density=Mini_Golf_Param.Wall.Density  ball_radius=Mini_Golf_Param.Ball.Radius  contact_k=Mini_Golf_Param.Wall.Stiffness  contact_b=Mini_Golf_Param.Wall.Damping  low_pass_filt_const=Mini_Golf_Param.Wall.Low_Pass_Filt_Const
  Ref : PMIOPort  Side=Right
  Ball : PMIOPort  Port=2  Side=Left
  connections:
  Spinning Wall/LConn2 -- Wall/LConn1
  Spinning Wall/RConn1 -- Wall/RConn1 -- Ball/RConn1
  Spinning Wall/LConn1 -- Ref/RConn1

== system Course_Holes_Lib/Course/Hole 6/Spinning X ==
  Spinning Wall : Golf_Components_Lib/Spinning Wall  length=Mini_Golf_Param.Hole_6.Wall_Obst1.Length  angle=Mini_Golf_Param.Hole_6.Wall_Obst1.Angle  offset=Mini_Golf_Param.Hole_6.Wall_Obst1.Offset  ang_spd=Mini_Golf_Param.Hole_6.Obst_Pin.Speed  height=Mini_Golf_Param.Ball.Radius*2  width=Mini_Golf_Param.Wall.Width  wall_density=Mini_Golf_Param.Wall.Density  ball_radius=Mini_Golf_Param.Ball.Radius  contact_k=Mini_Golf_Param.Wall.Stiffness  contact_b=Mini_Golf_Param.Wall.Damping  low_pass_filt_const=Mini_Golf_Param.Wall.Low_Pass_Filt_Const
  Wall : Golf_Components_Lib/Wall  length=Mini_Golf_Param.Hole_6.Wall_Obst2.Length  angle=Mini_Golf_Param.Hole_6.Wall_Obst2.Angle  offset=Mini_Golf_Param.Hole_6.Wall_Obst2.Offset*0  height=Mini_Golf_Param.Ball.Radius*2  width=Mini_Golf_Param.Wall.Width  wall_density=Mini_Golf_Param.Wall.Density  ball_radius=Mini_Golf_Param.Ball.Radius  contact_k=Mini_Golf_Param.Wall.Stiffness  contact_b=Mini_Golf_Param.Wall.Damping  low_pass_filt_const=Mini_Golf_Param.Wall.Low_Pass_Filt_Const
  Ref : PMIOPort  Side=Right
  Ball : PMIOPort  Port=2  Side=Left
  connections:
  Spinning Wall/LConn2 -- Wall/LConn1
  Wall/RConn1 -- Ball/RConn1 -- Spinning Wall/RConn1
  Spinning Wall/LConn1 -- Ref/RConn1

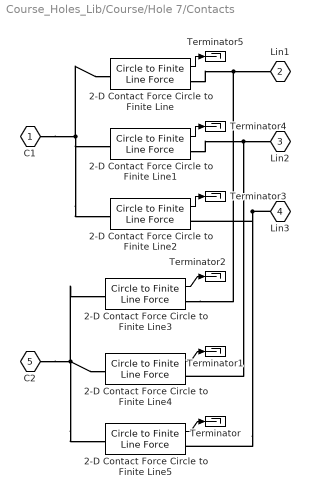
== system Course_Holes_Lib/Course/Hole 7/Contacts ==
  2-D Contact Force Circle to Finite Line : Contact_Forces_Lib/2D/Circle to Finite Line Force  circle_rad=Mini_Golf_Param.Ball.Radius  line_depth=Mini_Golf_Param.Wall.Width/2  line_length=Mini_Golf_Param.Hole_7.Wall_Right.Length  force_law=Linear  k_contact=Mini_Golf_Param.Wall.Stiffness  b_contact=Mini_Golf_Param.Wall.Damping  pen_full_damp_F=1e-4  pen_exponent=1  custom_param_1=1  custom_param_2=1  friction_law=None  mu_kinetic=0.5  mu_static=0.7  v_thr=0.001  vis_on=off  vis_opc_en=0  vis_len_linBz=0.1  vis_len_linBx=0.005  vis_len_cirFz=0.1  vis_len_cirFx=0.005  vis_clr=[0.9 0.2 0.2]  vis_opc=0.7
      settings: SourceProductName=Simscape Multibody Contact Forces Library
  2-D Contact Force Circle to Finite Line1 : Contact_Forces_Lib/2D/Circle to Finite Line Force  circle_rad=Mini_Golf_Param.Ball.Radius  line_depth=Mini_Golf_Param.Wall.Width/2  line_length=Mini_Golf_Param.Hole_7.Wall_Back.Length  force_law=Linear  k_contact=Mini_Golf_Param.Wall.Stiffness  b_contact=Mini_Golf_Param.Wall.Damping  pen_full_damp_F=1e-4  pen_exponent=1  custom_param_1=1  custom_param_2=1  friction_law=None  mu_kinetic=0.5  mu_static=0.7  v_thr=0.001  vis_on=off  vis_opc_en=0  vis_len_linBz=0.1  vis_len_linBx=0.005  vis_len_cirFz=0.1  vis_len_cirFx=0.005  vis_clr=[0.9 0.2 0.2]  vis_opc=0.7
      settings: SourceProductName=Simscape Multibody Contact Forces Library
  2-D Contact Force Circle to Finite Line2 : Contact_Forces_Lib/2D/Circle to Finite Line Force  circle_rad=Mini_Golf_Param.Ball.Radius  line_depth=Mini_Golf_Param.Wall.Width/2  line_length=Mini_Golf_Param.Hole_2.Wall_Right.Length  force_law=Linear  k_contact=Mini_Golf_Param.Wall.Stiffness  b_contact=Mini_Golf_Param.Wall.Damping  pen_full_damp_F=1e-4  pen_exponent=1  custom_param_1=1  custom_param_2=1  friction_law=None  mu_kinetic=0.5  mu_static=0.7  v_thr=0.001  vis_on=off  vis_opc_en=0  vis_len_linBz=0.1  vis_len_linBx=0.005  vis_len_cirFz=0.1  vis_len_cirFx=0.005  vis_clr=[0.9 0.2 0.2]  vis_opc=0.7
      settings: SourceProductName=Simscape Multibody Contact Forces Library
  2-D Contact Force Circle to Finite Line3 : Contact_Forces_Lib/2D/Circle to Finite Line Force  circle_rad=Mini_Golf_Param.Ball.Radius  line_depth=Mini_Golf_Param.Wall.Width/2  line_length=Mini_Golf_Param.Hole_7.Wall_Right.Length  force_law=Linear  k_contact=Mini_Golf_Param.Wall.Stiffness  b_contact=Mini_Golf_Param.Wall.Damping  pen_full_damp_F=1e-4  pen_exponent=1  custom_param_1=1  custom_param_2=1  friction_law=None  mu_kinetic=0.5  mu_static=0.7  v_thr=0.001  vis_on=off  vis_opc_en=0  vis_len_linBz=0.1  vis_len_linBx=0.005  vis_len_cirFz=0.1  vis_len_cirFx=0.005  vis_clr=[0.9 0.2 0.2]  vis_opc=0.7
      settings: SourceProductName=Simscape Multibody Contact Forces Library
  2-D Contact Force Circle to Finite Line4 : Contact_Forces_Lib/2D/Circle to Finite Line Force  circle_rad=Mini_Golf_Param.Ball.Radius  line_depth=Mini_Golf_Param.Wall.Width/2  line_length=Mini_Golf_Param.Hole_7.Wall_Back.Length  force_law=Linear  k_contact=Mini_Golf_Param.Wall.Stiffness  b_contact=Mini_Golf_Param.Wall.Damping  pen_full_damp_F=1e-4  pen_exponent=1  custom_param_1=1  custom_param_2=1  friction_law=None  mu_kinetic=0.5  mu_static=0.7  v_thr=0.001  vis_on=off  vis_opc_en=0  vis_len_linBz=0.1  vis_len_linBx=0.005  vis_len_cirFz=0.1  vis_len_cirFx=0.005  vis_clr=[0.9 0.2 0.2]  vis_opc=0.7
      settings: SourceProductName=Simscape Multibody Contact Forces Library
  2-D Contact Force Circle to Finite Line5 : Contact_Forces_Lib/2D/Circle to Finite Line Force  circle_rad=Mini_Golf_Param.Ball.Radius  line_depth=Mini_Golf_Param.Wall.Width/2  line_length=Mini_Golf_Param.Hole_2.Wall_Right.Length  force_law=Linear  k_contact=Mini_Golf_Param.Wall.Stiffness  b_contact=Mini_Golf_Param.Wall.Damping  pen_full_damp_F=1e-4  pen_exponent=1  custom_param_1=1  custom_param_2=1  friction_law=None  mu_kinetic=0.5  mu_static=0.7  v_thr=0.001  vis_on=off  vis_opc_en=0  vis_len_linBz=0.1  vis_len_linBx=0.005  vis_len_cirFz=0.1  vis_len_cirFx=0.005  vis_clr=[0.9 0.2 0.2]  vis_opc=0.7
      settings: SourceProductName=Simscape Multibody Contact Forces Library
  Terminator{,1..5} (6 alike) : Terminator
  C1 : PMIOPort  Side=Left
  Lin1 : PMIOPort  Port=2  Side=Right
  Lin2 : PMIOPort  Port=3  Side=Right
  Lin3 : PMIOPort  Port=4  Side=Right
  C2 : PMIOPort  Port=5  Side=Left
  wires:
  2-D Contact Force Circle to Finite Line5/1 -> Terminator/1
  2-D Contact Force Circle to Finite Line4/1 -> Terminator1/1
  2-D Contact Force Circle to Finite Line3/1 -> Terminator2/1
  2-D Contact Force Circle to Finite Line2/1 -> Terminator3/1
  2-D Contact Force Circle to Finite Line1/1 -> Terminator4/1
  2-D Contact Force Circle to Finite Line/1 -> Terminator5/1
  connections:
  2-D Contact Force Circle to Finite Line/LConn1 -- 2-D Contact Force Circle to Finite Line2/LConn1 -- C1/RConn1 -- 2-D Contact Force Circle to Finite Line1/LConn1
  2-D Contact Force Circle to Finite Line3/RConn1 -- 2-D Contact Force Circle to Finite Line/RConn1 -- Lin1/RConn1
  2-D Contact Force Circle to Finite Line1/RConn1 -- 2-D Contact Force Circle to Finite Line4/RConn1 -- Lin2/RConn1
  Lin3/RConn1 -- 2-D Contact Force Circle to Finite Line2/RConn1 -- 2-D Contact Force Circle to Finite Line5/RConn1
  2-D Contact Force Circle to Finite Line4/LConn1 -- 2-D Contact Force Circle to Finite Line3/LConn1 -- 2-D Contact Force Circle to Finite Line5/LConn1 -- C2/RConn1

== system Course_Holes_Lib/Course/Hole 8/Sliding Wall1 ==
  Slider Crank : Golf_Components_Lib/Slider Crank  initial_crank_spd=Mini_Golf_Param.Hole_8.Wall_Obst1.Initial_Crank_Spd  initial_crank_ang=Mini_Golf_Param.Hole_8.Wall_Obst1.Initial_Crank_Angle  rod_pin_radius=Mini_Golf_Param.Slider_Crank.Rod_Pin.Radius  rod_pin_length=Mini_Golf_Param.Slider_Crank.Rod_Pin.Length  rod_pin_z_offset=Mini_Golf_Param.Slider_Crank.Rod_Pin.Z_Offset  rod_dims=Mini_Golf_Param.Slider_Crank.Rod.Dimensions  rod_z_offset=Mini_Golf_Param.Slider_Crank.Rod.Z_Offset  crank_pin_radius=Mini_Golf_Param.Slider_Crank.Crank_Pin.Radius  crank_pin_length=Mini_Golf_Param.Slider_Crank.Crank_Pin.Length  crank_radius=Mini_Golf_Param.Slider_Crank.Crank.Radius  crank_length=Mini_Golf_Param.Slider_Crank.Crank.Length  crank_z_offset=Mini_Golf_Param.Slider_Crank.Crank.Z_Offset  density=Mini_Golf_Param.Slider_Crank.Density
  Sliding Wall : Golf_Components_Lib/Sliding Wall  length=Mini_Golf_Param.Hole_8.Wall_Obst1.Length  angle=Mini_Golf_Param.Hole_8.Wall_Obst1.Angle  offset=Mini_Golf_Param.Hole_8.Wall_Obst1.Offset  height=Mini_Golf_Param.Ball.Radius*2  width=Mini_Golf_Param.Wall.Width  wall_density=Mini_Golf_Param.Wall.Density  ball_radius=Mini_Golf_Param.Ball.Radius  contact_k=Mini_Golf_Param.Wall.Stiffness  contact_b=Mini_Golf_Param.Wall.Damping  low_pass_filt_const=Mini_Golf_Param.Wall.Low_Pass_Filt_Const
  Ref : PMIOPort  Side=Left
  Ball : PMIOPort  Port=2  Side=Right
  connections:
  Slider Crank/RConn1 -- Sliding Wall/LConn3
  Sliding Wall/LConn2 -- Slider Crank/RConn2
  Ref/RConn1 -- Sliding Wall/LConn1
  Ball/RConn1 -- Sliding Wall/RConn1

== system Course_Holes_Lib/Course/Hole 8/Sliding Wall2 ==
  Slider Crank : Golf_Components_Lib/Slider Crank  initial_crank_spd=Mini_Golf_Param.Hole_8.Wall_Obst2.Initial_Crank_Spd  initial_crank_ang=Mini_Golf_Param.Hole_8.Wall_Obst2.Initial_Crank_Angle  rod_pin_radius=Mini_Golf_Param.Slider_Crank.Rod_Pin.Radius  rod_pin_length=Mini_Golf_Param.Slider_Crank.Rod_Pin.Length  rod_pin_z_offset=Mini_Golf_Param.Slider_Crank.Rod_Pin.Z_Offset  rod_dims=Mini_Golf_Param.Slider_Crank.Rod.Dimensions  rod_z_offset=Mini_Golf_Param.Slider_Crank.Rod.Z_Offset  crank_pin_radius=Mini_Golf_Param.Slider_Crank.Crank_Pin.Radius  crank_pin_length=Mini_Golf_Param.Slider_Crank.Crank_Pin.Length  crank_radius=Mini_Golf_Param.Slider_Crank.Crank.Radius  crank_length=Mini_Golf_Param.Slider_Crank.Crank.Length  crank_z_offset=Mini_Golf_Param.Slider_Crank.Crank.Z_Offset  density=Mini_Golf_Param.Slider_Crank.Density
  Sliding Wall : Golf_Components_Lib/Sliding Wall  length=Mini_Golf_Param.Hole_8.Wall_Obst2.Length  angle=Mini_Golf_Param.Hole_8.Wall_Obst2.Angle  offset=Mini_Golf_Param.Hole_8.Wall_Obst2.Offset  height=Mini_Golf_Param.Ball.Radius*2  width=Mini_Golf_Param.Wall.Width  wall_density=Mini_Golf_Param.Wall.Density  ball_radius=Mini_Golf_Param.Ball.Radius  contact_k=Mini_Golf_Param.Wall.Stiffness  contact_b=Mini_Golf_Param.Wall.Damping  low_pass_filt_const=Mini_Golf_Param.Wall.Low_Pass_Filt_Const
  Ref : PMIOPort  Side=Left
  Ball : PMIOPort  Port=2  Side=Right
  connections:
  Ball/RConn1 -- Sliding Wall/RConn1
  Ref/RConn1 -- Sliding Wall/LConn1
  Sliding Wall/LConn2 -- Slider Crank/RConn2
  Slider Crank/RConn1 -- Sliding Wall/LConn3

== system Course_Holes_Lib/Course/Hole 8/Sliding Wall3 ==
  Slider Crank : Golf_Components_Lib/Slider Crank  initial_crank_spd=Mini_Golf_Param.Hole_8.Wall_Obst3.Initial_Crank_Spd  initial_crank_ang=Mini_Golf_Param.Hole_8.Wall_Obst3.Initial_Crank_Angle  rod_pin_radius=Mini_Golf_Param.Slider_Crank.Rod_Pin.Radius  rod_pin_length=Mini_Golf_Param.Slider_Crank.Rod_Pin.Length  rod_pin_z_offset=Mini_Golf_Param.Slider_Crank.Rod_Pin.Z_Offset  rod_dims=Mini_Golf_Param.Slider_Crank.Rod.Dimensions  rod_z_offset=Mini_Golf_Param.Slider_Crank.Rod.Z_Offset  crank_pin_radius=Mini_Golf_Param.Slider_Crank.Crank_Pin.Radius  crank_pin_length=Mini_Golf_Param.Slider_Crank.Crank_Pin.Length  crank_radius=Mini_Golf_Param.Slider_Crank.Crank.Radius  crank_length=Mini_Golf_Param.Slider_Crank.Crank.Length  crank_z_offset=Mini_Golf_Param.Slider_Crank.Crank.Z_Offset  density=Mini_Golf_Param.Slider_Crank.Density
  Sliding Wall : Golf_Components_Lib/Sliding Wall  length=Mini_Golf_Param.Hole_8.Wall_Obst3.Length  angle=Mini_Golf_Param.Hole_8.Wall_Obst3.Angle  offset=Mini_Golf_Param.Hole_8.Wall_Obst3.Offset  height=Mini_Golf_Param.Ball.Radius*2  width=Mini_Golf_Param.Wall.Width  wall_density=Mini_Golf_Param.Wall.Density  ball_radius=Mini_Golf_Param.Ball.Radius  contact_k=Mini_Golf_Param.Wall.Stiffness  contact_b=Mini_Golf_Param.Wall.Damping  low_pass_filt_const=Mini_Golf_Param.Wall.Low_Pass_Filt_Const
  Ref : PMIOPort  Side=Left
  Ball : PMIOPort  Port=2  Side=Right
  connections:
  Slider Crank/RConn1 -- Sliding Wall/LConn3
  Sliding Wall/LConn2 -- Slider Crank/RConn2
  Ref/RConn1 -- Sliding Wall/LConn1
  Ball/RConn1 -- Sliding Wall/RConn1
